simulink model "bike_model_v1_20190513_oldmodel"  (R2016b)
settings: Solver=ode23s  StartTime=0.0  StopTime=sim_time  FixedStep=Ts_IMU  MaxStep=Ts  RelTol=1e-3
values from neighbouring files (symbols this model uses):
  A = [0      0            1 ... (first row only)    [bike_init_v1_20190523_oldmodel_NOfeedback_RealModelComparison.m]    (also in bike_init_v1_20190524_oldmodel_positionfeedback_Nobalancing.m; bike_init_v1_20190527_oldmodel_NObalancing.m; bike_init_v1_20190527_oldmodel_positionfeedback_and_indicator.m; bike_init_v1_20190528_oldmodel_positionfeedback_and_indicator.m)
  B = [0; 1; (a_real*v*sin(lambda_real))/(h_real*b_real)]    [bike_init_v1_20190523_oldmodel_NOfeedback_RealModelComparison.m]    (also in bike_init_v1_20190524_oldmodel_positionfeedback_Nobalancing.m; bike_init_v1_20190527_oldmodel_NObalancing.m; bike_init_v1_20190527_oldmodel_positionfeedback_and_indicator.m; bike_init_v1_20190528_oldmodel_positionfeedback_and_indicator.m)
  b_model = 1.095*(1+(-0.1+(0.2*rand)))    [bike_init_v1_20190523_oldmodel_NOfeedback_RealModelComparison.m]    (also in bike_init_v1_20190524_oldmodel_positionfeedback_Nobalancing.m = 1.095; bike_init_v1_20190527_oldmodel_NObalancing.m = 1.095; bike_init_v1_20190527_oldmodel_positionfeedback_and_indicator.m = 1.095; bike_init_v1_20190528_oldmodel_positionfeedback_and_indicator.m = 1.095)
  b_real = 1.095    [bike_init_v1_20190523_oldmodel_NOfeedback_RealModelComparison.m]    (also in bike_init_v1_20190524_oldmodel_positionfeedback_Nobalancing.m; bike_init_v1_20190527_oldmodel_NObalancing.m; bike_init_v1_20190527_oldmodel_positionfeedback_and_indicator.m; bike_init_v1_20190528_oldmodel_positionfeedback_and_indicator.m)
  complementary = 0.985    [bike_init_v1_20190523_oldmodel_NOfeedback_RealModelComparison.m]    (also in bike_init_v1_20190524_oldmodel_positionfeedback_Nobalancing.m; bike_init_v1_20190527_oldmodel_NObalancing.m; bike_init_v1_20190527_oldmodel_positionfeedback_and_indicator.m; bike_init_v1_20190528_oldmodel_positionfeedback_and_indicator.m)
  cumulative_dist_along_path = [0;cumsum(dist_from_vertex_to_vertex,1)]    [bike_init_v1_20190523_oldmodel_NOfeedback_RealModelComparison.m]    (also in bike_init_v1_20190524_oldmodel_positionfeedback_Nobalancing.m; bike_init_v1_20190527_oldmodel_NObalancing.m; bike_init_v1_20190527_oldmodel_positionfeedback_and_indicator.m; bike_init_v1_20190528_oldmodel_positionfeedback_and_indicator.m)
  damp = 0.4    [bike_init_v1_20190523_oldmodel_NOfeedback_RealModelComparison.m]    (also in bike_init_v1_20190524_oldmodel_positionfeedback_Nobalancing.m; bike_init_v1_20190527_oldmodel_NObalancing.m; bike_init_v1_20190527_oldmodel_positionfeedback_and_indicator.m; bike_init_v1_20190528_oldmodel_positionfeedback_and_indicator.m)
  Dead_Band = [0.055,-0.055,0.005]    [bike_init_v1_20190523_oldmodel_NOfeedback_RealModelComparison.m]    (also in bike_init_v1_20190524_oldmodel_positionfeedback_Nobalancing.m; bike_init_v1_20190527_oldmodel_NObalancing.m; bike_init_v1_20190527_oldmodel_positionfeedback_and_indicator.m; bike_init_v1_20190528_oldmodel_positionfeedback_and_indicator.m)
  delay = 0.045    [bike_init_v1_20190523_oldmodel_NOfeedback_RealModelComparison.m]    (also in bike_init_v1_20190524_oldmodel_positionfeedback_Nobalancing.m; bike_init_v1_20190527_oldmodel_NObalancing.m; bike_init_v1_20190527_oldmodel_positionfeedback_and_indicator.m; bike_init_v1_20190528_oldmodel_positionfeedback_and_indicator.m)
  delta_control = 1    [bike_init_v1_20190523_oldmodel_NOfeedback_RealModelComparison.m]    (also in bike_init_v1_20190524_oldmodel_positionfeedback_Nobalancing.m; bike_init_v1_20190527_oldmodel_NObalancing.m; bike_init_v1_20190527_oldmodel_positionfeedback_and_indicator.m; bike_init_v1_20190528_oldmodel_positionfeedback_and_indicator.m)
  direct_control = 1    [bike_init_v1_20190523_oldmodel_NOfeedback_RealModelComparison.m]    (also in bike_init_v1_20190524_oldmodel_positionfeedback_Nobalancing.m; bike_init_v1_20190527_oldmodel_NObalancing.m; bike_init_v1_20190527_oldmodel_positionfeedback_and_indicator.m; bike_init_v1_20190528_oldmodel_positionfeedback_and_indicator.m)
  filter_model = 1    [bike_init_v1_20190523_oldmodel_NOfeedback_RealModelComparison.m]    (also in bike_init_v1_20190524_oldmodel_positionfeedback_Nobalancing.m; bike_init_v1_20190527_oldmodel_NObalancing.m; bike_init_v1_20190527_oldmodel_positionfeedback_and_indicator.m; bike_init_v1_20190528_oldmodel_positionfeedback_and_indicator.m)
  forward_motor_dynamics = 0    [bike_init_v1_20190523_oldmodel_NOfeedback_RealModelComparison.m]    (also in bike_init_v1_20190524_oldmodel_positionfeedback_Nobalancing.m; bike_init_v1_20190527_oldmodel_NObalancing.m; bike_init_v1_20190527_oldmodel_positionfeedback_and_indicator.m; bike_init_v1_20190528_oldmodel_positionfeedback_and_indicator.m)
  fr_oscil = 1    [bike_init_v1_20190523_oldmodel_NOfeedback_RealModelComparison.m]    (also in bike_init_v1_20190524_oldmodel_positionfeedback_Nobalancing.m; bike_init_v1_20190527_oldmodel_NObalancing.m; bike_init_v1_20190527_oldmodel_positionfeedback_and_indicator.m; bike_init_v1_20190528_oldmodel_positionfeedback_and_indicator.m)
  g = 9.81    [bike_init_v1_20190523_oldmodel_NOfeedback_RealModelComparison.m]    (also in bike_init_v1_20190524_oldmodel_positionfeedback_Nobalancing.m; bike_init_v1_20190527_oldmodel_NObalancing.m; bike_init_v1_20190527_oldmodel_positionfeedback_and_indicator.m; bike_init_v1_20190528_oldmodel_positionfeedback_and_indicator.m)
  gain = 0.3    [bike_init_v1_20190523_oldmodel_NOfeedback_RealModelComparison.m]    (also in bike_init_v1_20190524_oldmodel_positionfeedback_Nobalancing.m; bike_init_v1_20190527_oldmodel_NObalancing.m; bike_init_v1_20190527_oldmodel_positionfeedback_and_indicator.m; bike_init_v1_20190528_oldmodel_positionfeedback_and_indicator.m)
  IMU_height_model = 0.45*(1+(-0.1+(0.2*rand)))    [bike_init_v1_20190523_oldmodel_NOfeedback_RealModelComparison.m]    (also in bike_init_v1_20190524_oldmodel_positionfeedback_Nobalancing.m = 0.45; bike_init_v1_20190527_oldmodel_NObalancing.m = 0.45; bike_init_v1_20190527_oldmodel_positionfeedback_and_indicator.m = 0.45; bike_init_v1_20190528_oldmodel_positionfeedback_and_indicator.m = 0.45)
  IMU_height_real = 0.45    [bike_init_v1_20190523_oldmodel_NOfeedback_RealModelComparison.m]    (also in bike_init_v1_20190524_oldmodel_positionfeedback_Nobalancing.m; bike_init_v1_20190527_oldmodel_NObalancing.m; bike_init_v1_20190527_oldmodel_positionfeedback_and_indicator.m; bike_init_v1_20190528_oldmodel_positionfeedback_and_indicator.m)
  initial_states = [deg2rad(0) deg2rad(0) deg2rad(0)]    [bike_init_v1_20190523_oldmodel_NOfeedback_RealModelComparison.m]    (also in bike_init_v1_20190524_oldmodel_positionfeedback_Nobalancing.m; bike_init_v1_20190527_oldmodel_NObalancing.m; bike_init_v1_20190527_oldmodel_positionfeedback_and_indicator.m; bike_init_v1_20190528_oldmodel_positionfeedback_and_indicator.m = [deg2rad(1) deg2rad(0) deg2rad(0)])
  initial_x = path_x(1)+x_ini_diff    [bike_init_v1_20190523_oldmodel_NOfeedback_RealModelComparison.m]    (also in bike_init_v1_20190524_oldmodel_positionfeedback_Nobalancing.m; bike_init_v1_20190527_oldmodel_NObalancing.m; bike_init_v1_20190527_oldmodel_positionfeedback_and_indicator.m; bike_init_v1_20190528_oldmodel_positionfeedback_and_indicator.m)
  initial_y = radius+y_ini_diff    (= 20)    [bike_init_v1_20190523_oldmodel_NOfeedback_RealModelComparison.m]    (also in bike_init_v1_20190524_oldmodel_positionfeedback_Nobalancing.m; bike_init_v1_20190527_oldmodel_NObalancing.m; bike_init_v1_20190527_oldmodel_positionfeedback_and_indicator.m; bike_init_v1_20190528_oldmodel_positionfeedback_and_indicator.m)
  input_velocity = 2    [bike_init_v1_20190523_oldmodel_NOfeedback_RealModelComparison.m]    (also in bike_init_v1_20190524_oldmodel_positionfeedback_Nobalancing.m = 2.5; bike_init_v1_20190527_oldmodel_NObalancing.m = 2.5; bike_init_v1_20190527_oldmodel_positionfeedback_and_indicator.m = 3; bike_init_v1_20190528_oldmodel_positionfeedback_and_indicator.m = 7)
  K_full_dis = zeros(length(velocity_lqr),3)    [bike_init_v1_20190523_oldmodel_NOfeedback_RealModelComparison.m]    (also in bike_init_v1_20190524_oldmodel_positionfeedback_Nobalancing.m; bike_init_v1_20190527_oldmodel_NObalancing.m; bike_init_v1_20190527_oldmodel_positionfeedback_and_indicator.m; bike_init_v1_20190528_oldmodel_positionfeedback_and_indicator.m)
  lambda_model = deg2rad(70)*(1+(-0.1+(0.2*rand)))    [bike_init_v1_20190523_oldmodel_NOfeedback_RealModelComparison.m]    (also in bike_init_v1_20190524_oldmodel_positionfeedback_Nobalancing.m = deg2rad(70); bike_init_v1_20190527_oldmodel_NObalancing.m = deg2rad(70); bike_init_v1_20190527_oldmodel_positionfeedback_and_indicator.m = deg2rad(70); bike_init_v1_20190528_oldmodel_positionfeedback_and_indicator.m = deg2rad(70))
  lambda_real = deg2rad(70)    [bike_init_v1_20190523_oldmodel_NOfeedback_RealModelComparison.m]    (also in bike_init_v1_20190524_oldmodel_positionfeedback_Nobalancing.m; bike_init_v1_20190527_oldmodel_NObalancing.m; bike_init_v1_20190527_oldmodel_positionfeedback_and_indicator.m; bike_init_v1_20190528_oldmodel_positionfeedback_and_indicator.m)
  lat_control = 1    [bike_init_v1_20190523_oldmodel_NOfeedback_RealModelComparison.m]    (also in bike_init_v1_20190524_oldmodel_positionfeedback_Nobalancing.m; bike_init_v1_20190527_oldmodel_NObalancing.m; bike_init_v1_20190527_oldmodel_positionfeedback_and_indicator.m; bike_init_v1_20190528_oldmodel_positionfeedback_and_indicator.m)
  look_ahead = 0    [bike_init_v1_20190523_oldmodel_NOfeedback_RealModelComparison.m]    (also in bike_init_v1_20190524_oldmodel_positionfeedback_Nobalancing.m; bike_init_v1_20190527_oldmodel_NObalancing.m; bike_init_v1_20190527_oldmodel_positionfeedback_and_indicator.m; bike_init_v1_20190528_oldmodel_positionfeedback_and_indicator.m)
  max_handlebar = 40*(pi/180)    (= 0.698131700798)    [bike_init_v1_20190523_oldmodel_NOfeedback_RealModelComparison.m]    (also in bike_init_v1_20190524_oldmodel_positionfeedback_Nobalancing.m; bike_init_v1_20190527_oldmodel_NObalancing.m; bike_init_v1_20190527_oldmodel_positionfeedback_and_indicator.m; bike_init_v1_20190528_oldmodel_positionfeedback_and_indicator.m)
  max_roll = pi/2    (= 1.57079632679)    [bike_init_v1_20190523_oldmodel_NOfeedback_RealModelComparison.m]    (also in bike_init_v1_20190524_oldmodel_positionfeedback_Nobalancing.m; bike_init_v1_20190527_oldmodel_NObalancing.m; bike_init_v1_20190527_oldmodel_positionfeedback_and_indicator.m; bike_init_v1_20190528_oldmodel_positionfeedback_and_indicator.m)
  max_steering_motor_acc = inf    [bike_init_v1_20190523_oldmodel_NOfeedback_RealModelComparison.m]    (also in bike_init_v1_20190524_oldmodel_positionfeedback_Nobalancing.m; bike_init_v1_20190527_oldmodel_NObalancing.m; bike_init_v1_20190527_oldmodel_positionfeedback_and_indicator.m; bike_init_v1_20190528_oldmodel_positionfeedback_and_indicator.m)
  max_steering_motor_speed = 7.5    [bike_init_v1_20190523_oldmodel_NOfeedback_RealModelComparison.m]    (also in bike_init_v1_20190524_oldmodel_positionfeedback_Nobalancing.m; bike_init_v1_20190527_oldmodel_NObalancing.m; bike_init_v1_20190527_oldmodel_positionfeedback_and_indicator.m; bike_init_v1_20190528_oldmodel_positionfeedback_and_indicator.m)
  min_handlebar = -max_handlebar    (= -0.698131700798)    [bike_init_v1_20190523_oldmodel_NOfeedback_RealModelComparison.m]    (also in bike_init_v1_20190524_oldmodel_positionfeedback_Nobalancing.m; bike_init_v1_20190527_oldmodel_NObalancing.m; bike_init_v1_20190527_oldmodel_positionfeedback_and_indicator.m; bike_init_v1_20190528_oldmodel_positionfeedback_and_indicator.m)
  min_roll = - max_roll    (= -1.57079632679)    [bike_init_v1_20190523_oldmodel_NOfeedback_RealModelComparison.m]    (also in bike_init_v1_20190524_oldmodel_positionfeedback_Nobalancing.m; bike_init_v1_20190527_oldmodel_NObalancing.m; bike_init_v1_20190527_oldmodel_positionfeedback_and_indicator.m; bike_init_v1_20190528_oldmodel_positionfeedback_and_indicator.m)
  min_steering_motor_acc = -inf    [bike_init_v1_20190523_oldmodel_NOfeedback_RealModelComparison.m]    (also in bike_init_v1_20190524_oldmodel_positionfeedback_Nobalancing.m; bike_init_v1_20190527_oldmodel_NObalancing.m; bike_init_v1_20190527_oldmodel_positionfeedback_and_indicator.m; bike_init_v1_20190528_oldmodel_positionfeedback_and_indicator.m)
  min_steering_motor_speed = -7.5    [bike_init_v1_20190523_oldmodel_NOfeedback_RealModelComparison.m]    (also in bike_init_v1_20190524_oldmodel_positionfeedback_Nobalancing.m; bike_init_v1_20190527_oldmodel_NObalancing.m; bike_init_v1_20190527_oldmodel_positionfeedback_and_indicator.m; bike_init_v1_20190528_oldmodel_positionfeedback_and_indicator.m)
  noise = 1    [bike_init_v1_20190523_oldmodel_NOfeedback_RealModelComparison.m]    (also in bike_init_v1_20190524_oldmodel_positionfeedback_Nobalancing.m; bike_init_v1_20190527_oldmodel_NObalancing.m; bike_init_v1_20190527_oldmodel_positionfeedback_and_indicator.m; bike_init_v1_20190528_oldmodel_positionfeedback_and_indicator.m)
  noise_encoder = 1e-7    (= 1e-07)    [bike_init_v1_20190523_oldmodel_NOfeedback_RealModelComparison.m]    (also in bike_init_v1_20190524_oldmodel_positionfeedback_Nobalancing.m; bike_init_v1_20190527_oldmodel_NObalancing.m; bike_init_v1_20190527_oldmodel_positionfeedback_and_indicator.m; bike_init_v1_20190528_oldmodel_positionfeedback_and_indicator.m)
  noise_hall = 0    [bike_init_v1_20190523_oldmodel_NOfeedback_RealModelComparison.m]    (also in bike_init_v1_20190524_oldmodel_positionfeedback_Nobalancing.m = 0.01; bike_init_v1_20190527_oldmodel_NObalancing.m; bike_init_v1_20190527_oldmodel_positionfeedback_and_indicator.m = 0.01; bike_init_v1_20190528_oldmodel_positionfeedback_and_indicator.m = 0.01)
  oscillations_roll = 0    [bike_init_v1_20190523_oldmodel_NOfeedback_RealModelComparison.m]    (also in bike_init_v1_20190524_oldmodel_positionfeedback_Nobalancing.m; bike_init_v1_20190527_oldmodel_NObalancing.m; bike_init_v1_20190527_oldmodel_positionfeedback_and_indicator.m; bike_init_v1_20190528_oldmodel_positionfeedback_and_indicator.m)
  oscillations_steer = 0    [bike_init_v1_20190523_oldmodel_NOfeedback_RealModelComparison.m]    (also in bike_init_v1_20190524_oldmodel_positionfeedback_Nobalancing.m; bike_init_v1_20190527_oldmodel_NObalancing.m; bike_init_v1_20190527_oldmodel_positionfeedback_and_indicator.m; bike_init_v1_20190528_oldmodel_positionfeedback_and_indicator.m)
  parameters_model = [g h_model b_model a_model lambda_model c_model]    [bike_init_v1_20190523_oldmodel_NOfeedback_RealModelComparison.m]    (also in bike_init_v1_20190524_oldmodel_positionfeedback_Nobalancing.m; bike_init_v1_20190527_oldmodel_NObalancing.m; bike_init_v1_20190527_oldmodel_positionfeedback_and_indicator.m; bike_init_v1_20190528_oldmodel_positionfeedback_and_indicator.m)
  parameters_real = [g h_real b_real a_real lambda_real c_real]    [bike_init_v1_20190523_oldmodel_NOfeedback_RealModelComparison.m]    (also in bike_init_v1_20190524_oldmodel_positionfeedback_Nobalancing.m; bike_init_v1_20190527_oldmodel_NObalancing.m; bike_init_v1_20190527_oldmodel_positionfeedback_and_indicator.m; bike_init_v1_20190528_oldmodel_positionfeedback_and_indicator.m)
  path_tracking = 1    [bike_init_v1_20190523_oldmodel_NOfeedback_RealModelComparison.m]    (also in bike_init_v1_20190524_oldmodel_positionfeedback_Nobalancing.m; bike_init_v1_20190527_oldmodel_NObalancing.m; bike_init_v1_20190527_oldmodel_positionfeedback_and_indicator.m; bike_init_v1_20190528_oldmodel_positionfeedback_and_indicator.m = 0)
  path_x = [path_x1 path_x2 path_x3]    [bike_init_v1_20190523_oldmodel_NOfeedback_RealModelComparison.m]    (also in bike_init_v1_20190524_oldmodel_positionfeedback_Nobalancing.m; bike_init_v1_20190527_oldmodel_NObalancing.m; bike_init_v1_20190527_oldmodel_positionfeedback_and_indicator.m; bike_init_v1_20190528_oldmodel_positionfeedback_and_indicator.m)
  path_y = [path_y1 path_y2 path_y3]    [bike_init_v1_20190523_oldmodel_NOfeedback_RealModelComparison.m]    (also in bike_init_v1_20190524_oldmodel_positionfeedback_Nobalancing.m; bike_init_v1_20190527_oldmodel_NObalancing.m; bike_init_v1_20190527_oldmodel_positionfeedback_and_indicator.m; bike_init_v1_20190528_oldmodel_positionfeedback_and_indicator.m)
  plant_model = 1    [bike_init_v1_20190523_oldmodel_NOfeedback_RealModelComparison.m]    (also in bike_init_v1_20190524_oldmodel_positionfeedback_Nobalancing.m; bike_init_v1_20190527_oldmodel_NObalancing.m; bike_init_v1_20190527_oldmodel_positionfeedback_and_indicator.m; bike_init_v1_20190528_oldmodel_positionfeedback_and_indicator.m)
  roll_rate_coef = 0.9    [bike_init_v1_20190523_oldmodel_NOfeedback_RealModelComparison.m]    (also in bike_init_v1_20190524_oldmodel_positionfeedback_Nobalancing.m; bike_init_v1_20190527_oldmodel_NObalancing.m; bike_init_v1_20190527_oldmodel_positionfeedback_and_indicator.m; bike_init_v1_20190528_oldmodel_positionfeedback_and_indicator.m)
  sensordist = dout*pi/nrsensor    (= 0.439822971503)    [bike_init_v1_20190524_oldmodel_positionfeedback_Nobalancing.m]    (also in bike_init_v1_20190527_oldmodel_NObalancing.m; bike_init_v1_20190527_oldmodel_positionfeedback_and_indicator.m; bike_init_v1_20190528_oldmodel_positionfeedback_and_indicator.m; bike_init_v1_20190531_oldmodel_positionfeedback_and_indicator.m)
  steering_motor_limitations = 1    [bike_init_v1_20190523_oldmodel_NOfeedback_RealModelComparison.m]    (also in bike_init_v1_20190524_oldmodel_positionfeedback_Nobalancing.m; bike_init_v1_20190527_oldmodel_NObalancing.m; bike_init_v1_20190527_oldmodel_positionfeedback_and_indicator.m; bike_init_v1_20190528_oldmodel_positionfeedback_and_indicator.m)
  sys_con = ss(A,B,C,D)    [bike_init_v1_20190523_oldmodel_NOfeedback_RealModelComparison.m]    (also in bike_init_v1_20190524_oldmodel_positionfeedback_Nobalancing.m; bike_init_v1_20190527_oldmodel_NObalancing.m; bike_init_v1_20190527_oldmodel_positionfeedback_and_indicator.m; bike_init_v1_20190528_oldmodel_positionfeedback_and_indicator.m)
  sys_dis = c2d(sys_con,Ts)    [bike_init_v1_20190523_oldmodel_NOfeedback_RealModelComparison.m]    (also in bike_init_v1_20190524_oldmodel_positionfeedback_Nobalancing.m; bike_init_v1_20190527_oldmodel_NObalancing.m; bike_init_v1_20190527_oldmodel_positionfeedback_and_indicator.m; bike_init_v1_20190528_oldmodel_positionfeedback_and_indicator.m)
  ToleranceVelocityEst = 0.5    [bike_init_v1_20190524_oldmodel_positionfeedback_Nobalancing.m]    (also in bike_init_v1_20190527_oldmodel_NObalancing.m; bike_init_v1_20190527_oldmodel_positionfeedback_and_indicator.m; bike_init_v1_20190528_oldmodel_positionfeedback_and_indicator.m; bike_init_v1_20190531_oldmodel_positionfeedback_and_indicator.m)
  Ts = 0.04    [bike_init_v1_20190523_oldmodel_NOfeedback_RealModelComparison.m]    (also in bike_init_v1_20190524_oldmodel_positionfeedback_Nobalancing.m; bike_init_v1_20190527_oldmodel_NObalancing.m; bike_init_v1_20190527_oldmodel_positionfeedback_and_indicator.m; bike_init_v1_20190528_oldmodel_positionfeedback_and_indicator.m)
  Ts_IMU = 0.04    [bike_init_v1_20190523_oldmodel_NOfeedback_RealModelComparison.m]    (also in bike_init_v1_20190524_oldmodel_positionfeedback_Nobalancing.m; bike_init_v1_20190527_oldmodel_NObalancing.m; bike_init_v1_20190527_oldmodel_positionfeedback_and_indicator.m; bike_init_v1_20190528_oldmodel_positionfeedback_and_indicator.m)
  velocity_lqr = [velocity_lqr-0.1 velocity_lqr velocity_lqr+0.1]    [bike_init_v1_20190523_oldmodel_NOfeedback_RealModelComparison.m]    (also in bike_init_v1_20190524_oldmodel_positionfeedback_Nobalancing.m; bike_init_v1_20190527_oldmodel_NObalancing.m; bike_init_v1_20190527_oldmodel_positionfeedback_and_indicator.m; bike_init_v1_20190528_oldmodel_positionfeedback_and_indicator.m)
  velocity_wave_amp = 0.5    [bike_init_v1_20190523_oldmodel_NOfeedback_RealModelComparison.m]    (also in bike_init_v1_20190524_oldmodel_positionfeedback_Nobalancing.m; bike_init_v1_20190527_oldmodel_NObalancing.m; bike_init_v1_20190527_oldmodel_positionfeedback_and_indicator.m; bike_init_v1_20190528_oldmodel_positionfeedback_and_indicator.m)
  velocity_wave_freq = 0.3*2*pi    (= 1.88495559215)    [bike_init_v1_20190523_oldmodel_NOfeedback_RealModelComparison.m]    (also in bike_init_v1_20190524_oldmodel_positionfeedback_Nobalancing.m; bike_init_v1_20190527_oldmodel_NObalancing.m; bike_init_v1_20190527_oldmodel_positionfeedback_and_indicator.m; bike_init_v1_20190528_oldmodel_positionfeedback_and_indicator.m)
undefined symbols (not defined in the file or in its folder): curvature
libraries: simulink x13, dspsigops x2, simulink_extras x1
(part 2 of 3)

== system bike_model_v1_20190513_oldmodel/Balance Controller/LQR Controller ==
  note: Input = steering angular velocity
  Velocity : Inport
  State Error : Inport  Port=2
  1-D Lookup Table : Lookup_n-D  NumberOfTableDimensions=1  BreakpointsForDimension1=velocity_lqr  BreakpointsForDimension2=velocity_lqr  BreakpointsForDimension3=velocity_lqr  BreakpointsForDimension4=velocity_lqr  Table=K_full_dis(:,1)  InternalRulePriority=Speed  RndMeth=Simplest  InputSameDT=on
  1-D Lookup Table1 : Lookup_n-D  NumberOfTableDimensions=1  BreakpointsForDimension1=velocity_lqr  BreakpointsForDimension2=velocity_lqr  BreakpointsForDimension3=velocity_lqr  BreakpointsForDimension4=velocity_lqr  Table=K_full_dis(:,2)  InternalRulePriority=Speed  RndMeth=Simplest  InputSameDT=on
  1-D Lookup Table2 : Lookup_n-D  NumberOfTableDimensions=1  BreakpointsForDimension1=velocity_lqr  BreakpointsForDimension2=velocity_lqr  BreakpointsForDimension3=velocity_lqr  BreakpointsForDimension4=velocity_lqr  Table=K_full_dis(:,3)  InternalRulePriority=Speed  RndMeth=Simplest  InputSameDT=on
  Display1 : Display
  Mux : Mux  Inputs=3
  Product : Product  Multiplication=Matrix(*)
  Scope : Scope
  Transpose : Math  Operator=transpose  SaturateOnIntegerOverflow=on
  Zero-Order Hold : ZeroOrderHold  SampleTime=Ts
  Zero-Order Hold1 : ZeroOrderHold  SampleTime=Ts
  Calculated Input : Outport
  wires:
  1-D Lookup Table/1 -> Mux/1  "K1"
  1-D Lookup Table1/1 -> Mux/2  "K2"
  State Error/1 -> Zero-Order Hold1/1
  Product/1 -> Zero-Order Hold/1
  1-D Lookup Table2/1 -> Mux/3  "K3"
  Velocity/1 -> 1-D Lookup Table2/1, 1-D Lookup Table1/1, 1-D Lookup Table/1
  Mux/1 -> Product/2, Display1/1
  Transpose/1 -> Product/1
  Zero-Order Hold/1 -> Calculated Input/1
  Zero-Order Hold1/1 -> Scope/1, Transpose/1

== system bike_model_v1_20190513_oldmodel/Balance Controller/Reference States ==
  Velocity : Inport
  Delta Ref : Inport  Port=2
  Bike Parameters : Constant  Value=parameters_real
  Constant : Constant  Value=path_tracking
  Mux5 : Mux  Inputs=3
  Reference Roll Angle Calculator : MATLAB Function  TreatAsAtomicUnit=on
  Switch : Switch  Criteria=u2 > Threshold
  Reference States : Outport
  wires:
  Bike Parameters/1 -> Reference Roll Angle Calculator/1(parameters_real)
  Switch/1 -> Mux5/2, Reference Roll Angle Calculator/3(delta_ref)
  Reference Roll Angle Calculator/1(phi_ref) -> Mux5/1
  Velocity/1 -> Reference Roll Angle Calculator/2(velocity)
  Mux5/1 -> Reference States/1
  Constant/1 -> Switch/2
  Delta Ref/1 -> Switch/1

== system bike_model_v1_20190513_oldmodel/Complementary filter/Complementary Filter ==
  Roll Angle Estimation due to Accelerometer : Inport
  Roll Rate due to Gyroscope : Inport  Port=2
  Delay : Delay  DelayLength=1  InitialCondition=0
  Gain2 : Gain  Gain=complementary
  Gain3 : Gain  Gain=1-complementary
  Gain4 : Gain  Gain=Ts_IMU
  Sum3 : Sum  Inputs=|++
  Sum4 : Sum  Inputs=++|
  Roll Angle Estimation : Outport
  wires:
  Roll Angle Estimation due to Accelerometer/1 -> Gain3/1  "Roll_acc"
  Sum3/1 -> Gain2/1
  Roll Rate due to Gyroscope/1 -> Gain4/1
  Delay/1 -> Sum3/2
  Gain4/1 -> Sum3/1
  Gain2/1 -> Sum4/2
  Gain3/1 -> Sum4/1
  Sum4/1 -> Delay/1, Roll Angle Estimation/1

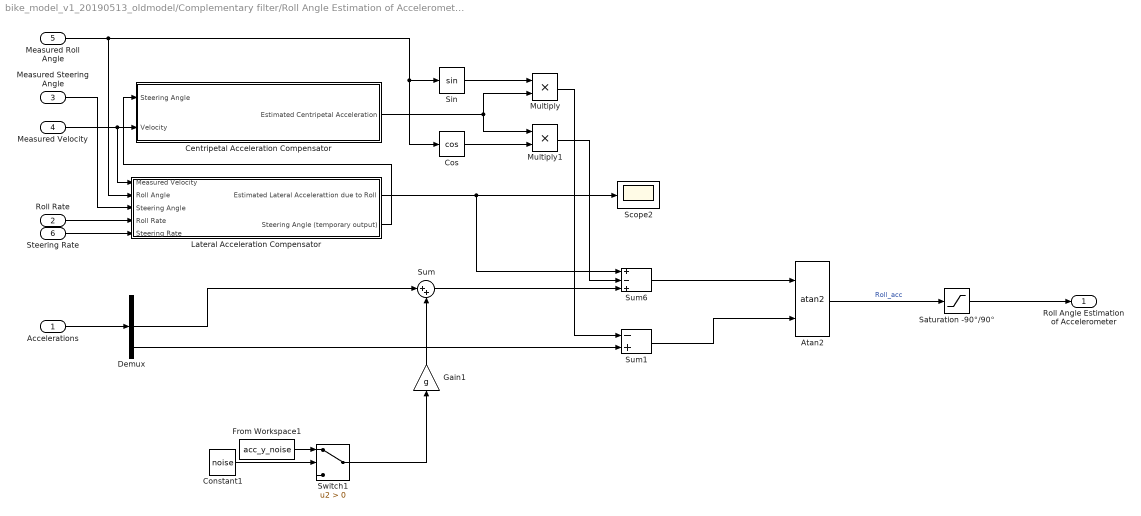
== system bike_model_v1_20190513_oldmodel/Complementary filter/Roll Angle Estimation of Accelerometer ==
  Accelerations : Inport
  Roll Rate : Inport  Port=2
  Measured Steering Angle : Inport  Port=3
  Measured Velocity : Inport  Port=4
  Measured Roll Angle : Inport  Port=5
  Steering Rate : Inport  Port=6
  Atan2 : Trigonometry  Operator=atan2
  Centripetal Acceleration Compensator : Subsystem
  Constant1 : Constant  Value=noise
  Cos : Trigonometry  Operator=cos
  Demux : Demux  Outputs=3
  From Workspace1 : FromWorkspace  VariableName=acc_y_noise  SampleTime=0
  Gain1 : Gain  Gain=g
  Lateral Acceleration Compensator : Subsystem
  Multiply : Product
  Multiply1 : Product
  Saturation -90°/90° : Saturate  UpperLimit=max_roll  LowerLimit=min_roll
  Scope2 : Scope
  Sin : Trigonometry
  Sum : Sum  Inputs=|++
  Sum1 : Sum  Inputs=-+
  Sum6 : Sum  Inputs=+-+
  Switch1 : Switch  Criteria=u2 > Threshold
  Roll Angle Estimation of Accelerometer : Outport
  wires:
  Sum1/1 -> Atan2/2
  Lateral Acceleration Compensator/1(Estimated Lateral Accelerattion due to Roll) -> Scope2/1, Sum6/1
  Atan2/1 -> Saturation -90°/90°/1  "Roll_acc"
  Roll Rate/1 -> Lateral Acceleration Compensator/4(Roll Rate)
  Demux/2 -> Sum/1
  Accelerations/1 -> Demux/1
  Measured Velocity/1 -> Lateral Acceleration Compensator/1(Measured Velocity), Centripetal Acceleration Compensator/2(Velocity)
  Measured Steering Angle/1 -> Lateral Acceleration Compensator/3(Steering Angle)
  Centripetal Acceleration Compensator/1(Estimated Centripetal Acceleration) -> Multiply/2, Multiply1/1
  Measured Roll Angle/1 -> Lateral Acceleration Compensator/2(Roll Angle), Sin/1, Cos/1
  Cos/1 -> Multiply1/2
  Sin/1 -> Multiply/1
  Multiply1/1 -> Sum6/2
  Demux/3 -> Sum1/2
  Multiply/1 -> Sum1/1
  Steering Rate/1 -> Lateral Acceleration Compensator/5(Steering Rate)
  Sum6/1 -> Atan2/1
  Lateral Acceleration Compensator/2(Steering Angle (temporary output)) -> Centripetal Acceleration Compensator/1(Steering Angle)
  From Workspace1/1 -> Switch1/1
  Constant1/1 -> Switch1/2
  Sum/1 -> Sum6/3
  Switch1/1 -> Gain1/1
  Gain1/1 -> Sum/2
  Saturation -90°/90°/1 -> Roll Angle Estimation of Accelerometer/1

== system bike_model_v1_20190513_oldmodel/Global Angles and Coordinates Calculator/Measured Bike Angles to Global Angles ==
  Velocity : Inport
  Steering Angle : Inport  Port=2
  Gain : Gain  Gain=1/b_model
  Integrator : Integrator
  MATLAB Function : MATLAB Function  TreatAsAtomicUnit=on
  Multiply : Product
  Parameters : Constant  Value=parameters_model
  Scope : Scope  NumInputPorts=2
  Tan : Trigonometry  Operator=tan
  psi : Outport
  beta : Outport  Port=2
  wires:
  Integrator/1 -> psi/1
  MATLAB Function/1(psi_d) -> Scope/1, Integrator/1
  Steering Angle/1 -> Tan/1, MATLAB Function/3(delta)
  Parameters/1 -> MATLAB Function/2(parameters_model)
  Velocity/1 -> Multiply/1, MATLAB Function/1(v)
  MATLAB Function/2(beta) -> beta/1
  Tan/1 -> Multiply/2
  Multiply/1 -> Gain/1
  Gain/1 -> Scope/2

== system bike_model_v1_20190513_oldmodel/Global Angles and Coordinates Calculator/Measured Global Angles to Global Coordinates ==
  Velocity : Inport
  Psi : Inport  Port=2
  Beta : Inport  Port=3
  Constant : Constant  Value=initial_y
  Constant1 : Constant  Value=initial_x
  Integrator1 : Integrator
  Integrator2 : Integrator
  MATLAB Function1 : MATLAB Function  TreatAsAtomicUnit=on
  Mux : Mux  Inputs=2
  Sum : Sum  Inputs=|++
  Sum1 : Sum  Inputs=++|
  "Position (X, Y)" : Outport
  wires:
  MATLAB Function1/2(Ydot) -> Integrator2/1  "Ydot"
  MATLAB Function1/1(Xdot) -> Integrator1/1  "Xdot"
  Psi/1 -> MATLAB Function1/2(psi)
  Beta/1 -> MATLAB Function1/3(beta)
  Velocity/1 -> MATLAB Function1/1(v)
  Integrator2/1 -> Sum/1
  Constant/1 -> Sum/2
  Sum/1 -> Mux/2
  Integrator1/1 -> Sum1/2
  Sum1/1 -> Mux/1
  Constant1/1 -> Sum1/1
  Mux/1 -> "Position (X, Y)"/1

== system bike_model_v1_20190513_oldmodel/Global Angles and Coordinates Calculator/Path Plotter Reality ==
  Position : Inport
  Demux : Demux  Outputs=2
  To Workspace : ToWorkspace  VariableName=X_BIKE  SaveFormat=Timeseries  SampleTime=Ts
  To Workspace1 : ToWorkspace  VariableName=Y_BIKE  SaveFormat=Timeseries  SampleTime=Ts
  XY Graph : simulink/Sinks/XY Graph  Commented=on  xmin=min(path_x)-5  xmax=max(path_x)+5  ymin=min(path_y)-5  ymax=max(path_y)+5  st=-1
  wires:
  Demux/1 -> XY Graph/1, To Workspace/1  "X"
  Demux/2 -> XY Graph/2, To Workspace1/1  "Y"
  Position/1 -> Demux/1

== system bike_model_v1_20190513_oldmodel/Global Angles and Coordinates Calculator/Path Plotter estimation ==
  Position : Inport
  Demux : Demux  Outputs=2
  To Workspace : ToWorkspace  VariableName=X_BIKE_estim  SaveFormat=Timeseries  SampleTime=Ts
  To Workspace1 : ToWorkspace  VariableName=Y_BIKE_estim  SaveFormat=Timeseries  SampleTime=Ts
  XY Graph : simulink/Sinks/XY Graph  Commented=on  xmin=min(path_x)-5  xmax=max(path_x)+5  ymin=min(path_y)-5  ymax=max(path_y)+5  st=-1
  wires:
  Demux/1 -> XY Graph/1, To Workspace/1  "X"
  Demux/2 -> XY Graph/2, To Workspace1/1  "Y"
  Position/1 -> Demux/1

== system bike_model_v1_20190513_oldmodel/Global Angles and Coordinates Calculator/True Bike Angles to Global Angles2 ==
  Velocity : Inport
  Steering Angle : Inport  Port=2
  Integrator : Integrator
  MATLAB Function : MATLAB Function  TreatAsAtomicUnit=on
  Real Bike Parameters : Constant  Value=parameters_real
  To Workspace6 : ToWorkspace  VariableName=PSI  SaveFormat=Timeseries  SampleTime=Ts
  To Workspace7 : ToWorkspace  VariableName=BETA  SaveFormat=Timeseries  SampleTime=Ts
  psi : Outport
  beta : Outport  Port=2
  wires:
  Integrator/1 -> To Workspace6/1, psi/1
  MATLAB Function/1(psi_d) -> Integrator/1
  Steering Angle/1 -> MATLAB Function/3(delta)
  Real Bike Parameters/1 -> MATLAB Function/2(parameters_real)
  Velocity/1 -> MATLAB Function/1(v)
  MATLAB Function/2(beta) -> beta/1, To Workspace7/1

== system bike_model_v1_20190513_oldmodel/Global Angles and Coordinates Calculator/True Global Angles to Global Coordinates ==
  Velocity : Inport
  Psi : Inport  Port=2
  Beta : Inport  Port=3
  Constant : Constant  Value=initial_y
  Constant1 : Constant  Value=initial_x
  Integrator1 : Integrator
  Integrator2 : Integrator
  MATLAB Function1 : MATLAB Function  TreatAsAtomicUnit=on
  Mux : Mux  Inputs=2
  Sum : Sum  Inputs=|++
  Sum1 : Sum  Inputs=++|
  "Position (X, Y)" : Outport
  wires:
  MATLAB Function1/2(Ydot) -> Integrator2/1  "Ydot"
  MATLAB Function1/1(Xdot) -> Integrator1/1  "Xdot"
  Psi/1 -> MATLAB Function1/2(psi)
  Beta/1 -> MATLAB Function1/3(beta)
  Velocity/1 -> MATLAB Function1/1(v)
  Integrator2/1 -> Sum/1
  Constant/1 -> Sum/2
  Sum/1 -> Mux/2
  Integrator1/1 -> Sum1/2
  Sum1/1 -> Mux/1
  Constant1/1 -> Sum1/1
  Mux/1 -> "Position (X, Y)"/1

== system bike_model_v1_20190513_oldmodel/IMU/IMU ==
  Lateral Acceleration : Inport
  Centripetal Acceleration : Inport  Port=2
  True Velocity : Inport  Port=3
  True Roll Angle : Inport  Port=4
  Measured Steering Angle : Inport  Port=5
  IMU Accelerometer : Subsystem
  IMU Gyroscope : Subsystem
  Accelerations : Outport
  Roll Rates : Outport  Port=2
  wires:
  Lateral Acceleration/1 -> IMU Accelerometer/1(Lateral Acceleration of the IMU due to Roll)
  Centripetal Acceleration/1 -> IMU Accelerometer/2(Centripetal Acceleration due to Path Curvature)
  True Roll Angle/1 -> IMU Gyroscope/2(True Roll Angle), IMU Accelerometer/4(True Roll Angle)
  IMU Accelerometer/1(Accelerations) -> Accelerations/1
  IMU Gyroscope/1(Roll rates) -> Roll Rates/1
  True Velocity/1 -> IMU Gyroscope/1(True Velocity), IMU Accelerometer/3(True Velocity)
  Measured Steering Angle/1 -> IMU Gyroscope/3(Measured Steering Angle)

== system bike_model_v1_20190513_oldmodel/Path Tracking Controllers/Lateral Error ==
  Psi Sigma : Inport
  Position Error (X,Y) : Inport  Port=2
  Cos : Trigonometry  Operator=cos
  Demux : Demux  Outputs=2
  Product : Product
  Product1 : Product
  Sin : Trigonometry
  Sum : Sum  Inputs=+-|
  To Workspace4 : ToWorkspace  VariableName=LAT_ERR  SaveFormat=Timeseries  SampleTime=Ts
  Lateral Error : Outport
  wires:
  Cos/1 -> Product/2
  Sin/1 -> Product1/1
  Psi Sigma/1 -> Cos/1, Sin/1
  Product1/1 -> Sum/2
  Product/1 -> Sum/1
  Sum/1 -> To Workspace4/1, Lateral Error/1  "Lateral Error"
  Demux/1 -> Product1/2  "X Position Error"
  Demux/2 -> Product/1  "Y Position Error"
  Position Error (X,Y)/1 -> Demux/1

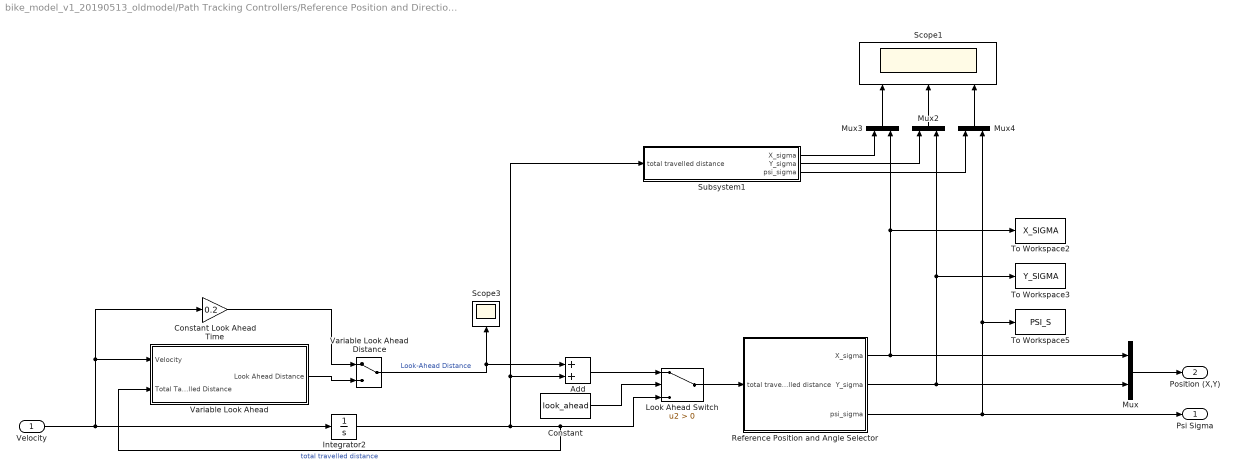
== system bike_model_v1_20190513_oldmodel/Path Tracking Controllers/Reference Position and Direction in Global CS with variable Look Ahead ==
  Velocity : Inport
  Add : Sum
  Constant : Constant  Value=look_ahead
  Constant Look Ahead Time : Gain  Gain=0.2
  Integrator2 : Integrator
  Look Ahead Switch : Switch  Criteria=u2 > Threshold
  Mux{,2..4} (4 alike) : Mux  Inputs=2
  Reference Position and Angle Selector : Subsystem
  Scope1 : Scope  NumInputPorts=3
  Scope3 : Scope
  Subsystem1 : Subsystem
  To Workspace2 : ToWorkspace  VariableName=X_SIGMA  SaveFormat=Timeseries  SampleTime=Ts
  To Workspace3 : ToWorkspace  VariableName=Y_SIGMA  SaveFormat=Timeseries  SampleTime=Ts
  To Workspace5 : ToWorkspace  VariableName=PSI_S  SaveFormat=Timeseries  SampleTime=Ts
  Variable Look Ahead Distance : ManualSwitch
  Variable Look Ahead : Subsystem
  Psi Sigma : Outport
  Position (X,Y) : Outport  Port=2
  wires:
  Constant Look Ahead Time/1 -> Variable Look Ahead Distance/1
  Reference Position and Angle Selector/3(psi_sigma) -> To Workspace5/1, Mux4/2, Psi Sigma/1
  Mux3/1 -> Scope1/1
  Subsystem1/3(psi_sigma) -> Mux4/1
  Mux2/1 -> Scope1/2
  Mux4/1 -> Scope1/3
  Velocity/1 -> Integrator2/1, Constant Look Ahead Time/1, Variable Look Ahead/1(Velocity)
  Add/1 -> Look Ahead Switch/1
  Reference Position and Angle Selector/2(Y_sigma) -> To Workspace3/1, Mux2/2, Mux/2
  Look Ahead Switch/1 -> Reference Position and Angle Selector/1(total travelled distance)
  Subsystem1/2(Y_sigma) -> Mux2/1
  Integrator2/1 -> Variable Look Ahead/2(Total Tavelled Distance), Look Ahead Switch/3, Subsystem1/1(total travelled distance), Add/2  "total travelled distance"
  Subsystem1/1(X_sigma) -> Mux3/1
  Reference Position and Angle Selector/1(X_sigma) -> Mux3/2, To Workspace2/1, Mux/1
  Variable Look Ahead Distance/1 -> Scope3/1, Add/1  "Look-Ahead Distance"
  Constant/1 -> Look Ahead Switch/2
  Mux/1 -> Position (X,Y)/1
  Variable Look Ahead/1(Look Ahead Distance) -> Variable Look Ahead Distance/2

== system bike_model_v1_20190513_oldmodel/Physical Bike/Centripetal Acceleration Calculator ==
  True Steering Angle : Inport
  True Velocity : Inport  Port=2
  Divide : Product  Inputs=*/
  Gain : Gain  Gain=sin(lambda_real)
  Multiply : Product
  Square : Math  Operator=square  SaturateOnIntegerOverflow=on
  Tan : Trigonometry  Operator=tan
  b Real Bike : Constant  Value=b_real
  Centripetal Acceleration : Outport
  wires:
  True Velocity/1 -> Square/1
  Square/1 -> Divide/1
  b Real Bike/1 -> Divide/2
  True Steering Angle/1 -> Gain/1
  Divide/1 -> Multiply/1
  Tan/1 -> Multiply/2
  Multiply/1 -> Centripetal Acceleration/1
  Gain/1 -> Tan/1

== system bike_model_v1_20190513_oldmodel/Physical Bike/Check Phi Limits ==
  x : Inport
  Roll Lower Bound : simulink/Model Verification/Check Static  Lower Bound  Description=min_roll <= u  min=min_roll  min_included=on  enabled=on  stopWhenAssertionFail=on  export=off  icon=graphic
  Roll Upper Bound : simulink/Model Verification/Check Static  Upper Bound  Description=u <= max_roll  max=max_roll  max_included=on  enabled=on  stopWhenAssertionFail=on  export=off  icon=graphic
  wires:
  x/1 -> Roll Lower Bound/1, Roll Upper Bound/1  "Roll Angle"

== system bike_model_v1_20190513_oldmodel/Physical Bike/Lateral Acceleration (due to Roll) Calculator ==
  Roll Acceleration : Inport
  Constant3 : Constant  Value=IMU_height_real
  Multiply : Product
  Lateral Acceleration : Outport
  wires:
  Multiply/1 -> Lateral Acceleration/1
  Constant3/1 -> Multiply/1
  Roll Acceleration/1 -> Multiply/2

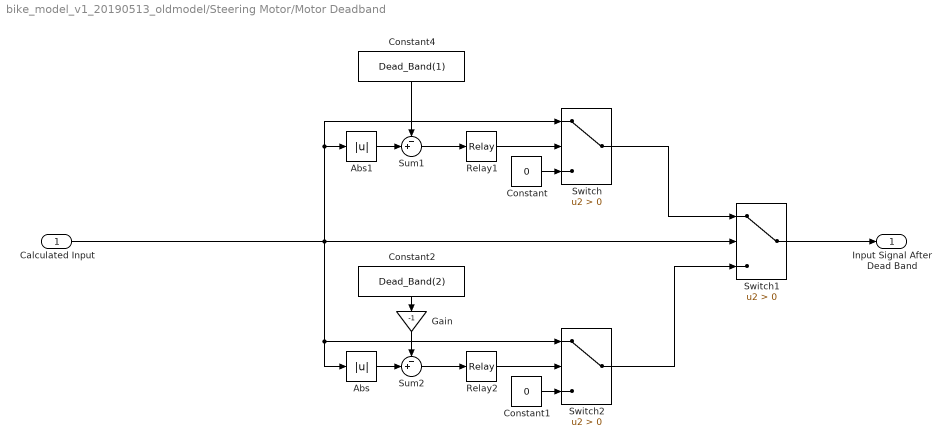
== system bike_model_v1_20190513_oldmodel/Steering Motor/Motor Deadband ==
  Calculated Input : Inport
  Abs : Abs
  Abs1 : Abs
  Constant : Constant  Value=0  SampleTime=Ts
  Constant1 : Constant  Value=0  SampleTime=Ts
  Constant2 : Constant  Value=Dead_Band(2)  SampleTime=Ts
  Constant4 : Constant  Value=Dead_Band(1)  SampleTime=Ts
  Gain : Gain  Gain=-1
  Relay1 : Relay  OnSwitchValue=Dead_Band(3)  OffSwitchValue=-Dead_Band(3)
  Relay2 : Relay  OnSwitchValue=Dead_Band(3)  OffSwitchValue=-Dead_Band(3)
  Sum1 : Sum  Inputs=-+|
  Sum2 : Sum  Inputs=-+|
  Switch : Switch  Criteria=u2 > Threshold
  Switch1 : Switch  Criteria=u2 > Threshold
  Switch2 : Switch  Criteria=u2 > Threshold
  Input Signal After Dead Band : Outport
  wires:
  Constant4/1 -> Sum1/1
  Sum1/1 -> Relay1/1
  Relay1/1 -> Switch/2
  Switch/1 -> Switch1/1
  Constant/1 -> Switch/3
  Switch1/1 -> Input Signal After Dead Band/1
  Switch2/1 -> Switch1/3
  Constant1/1 -> Switch2/3
  Gain/1 -> Sum2/1
  Calculated Input/1 -> Abs/1, Switch2/1, Abs1/1, Switch/1, Switch1/2
  Sum2/1 -> Relay2/1
  Relay2/1 -> Switch2/2
  Abs/1 -> Sum2/2
  Abs1/1 -> Sum1/2
  Constant2/1 -> Gain/1

== system bike_model_v1_20190513_oldmodel/Steering Motor/Velocity Saturation wrt Max and Min Handle Bar Angles ==
  Reference Velocity : Inport
  States : Inport  Port=2
  AND : Logic  IconShape=distinctive  AllPortsSameDT=off  OutDataTypeStr=boolean
  AND1 : Logic  IconShape=distinctive  AllPortsSameDT=off  OutDataTypeStr=boolean
  Compare To Constant : simulink/Logic and Bit Operations/Compare To Constant  relop=>=  const=max_handlebar  OutDataTypeStr=boolean
  Compare To Constant1 : simulink/Logic and Bit Operations/Compare To Constant  relop=<=  const=min_handlebar  OutDataTypeStr=boolean
  Compare To Zero : simulink/Logic and Bit Operations/Compare To Zero  relop=>=  OutDataTypeStr=boolean
  Compare To Zero1 : simulink/Logic and Bit Operations/Compare To Zero  relop=<=  OutDataTypeStr=boolean
  Constant : Constant  Value=0
  Demux : Demux  Outputs=3
  OR : Logic  Operator=OR  IconShape=distinctive  AllPortsSameDT=off  OutDataTypeStr=boolean
  Switch : Switch  Criteria=u2 > Threshold
  Output Steering Velocity : Outport
  wires:
  Switch/1 -> Output Steering Velocity/1
  Constant/1 -> Switch/1
  States/1 -> Demux/1
  Compare To Zero/1 -> AND/1
  Compare To Zero1/1 -> AND1/2
  Demux/2 -> Compare To Constant/1, Compare To Constant1/1
  Compare To Constant1/1 -> AND1/1
  AND/1 -> OR/1
  AND1/1 -> OR/2
  Compare To Constant/1 -> AND/2
  Reference Velocity/1 -> Compare To Zero1/1, Compare To Zero/1, Switch/3
  OR/1 -> Switch/2

== system bike_model_v1_20190513_oldmodel/Complementary filter/Roll Angle Estimation of Accelerometer/Centripetal Acceleration Compensator ==
  Steering Angle : Inport
  Velocity : Inport  Port=2
  Bike Model b : Constant  Value=b_model
  Divide : Product  Inputs=*/
  Gain : Gain  Gain=sin(lambda_model)
  Multiply : Product
  Square : Math  Operator=square  SaturateOnIntegerOverflow=on
  Tan : Trigonometry  Operator=tan
  Estimated Centripetal Acceleration : Outport
  wires:
  Velocity/1 -> Square/1
  Square/1 -> Divide/1
  Bike Model b/1 -> Divide/2
  Steering Angle/1 -> Gain/1
  Divide/1 -> Multiply/1
  Tan/1 -> Multiply/2
  Multiply/1 -> Estimated Centripetal Acceleration/1
  Gain/1 -> Tan/1

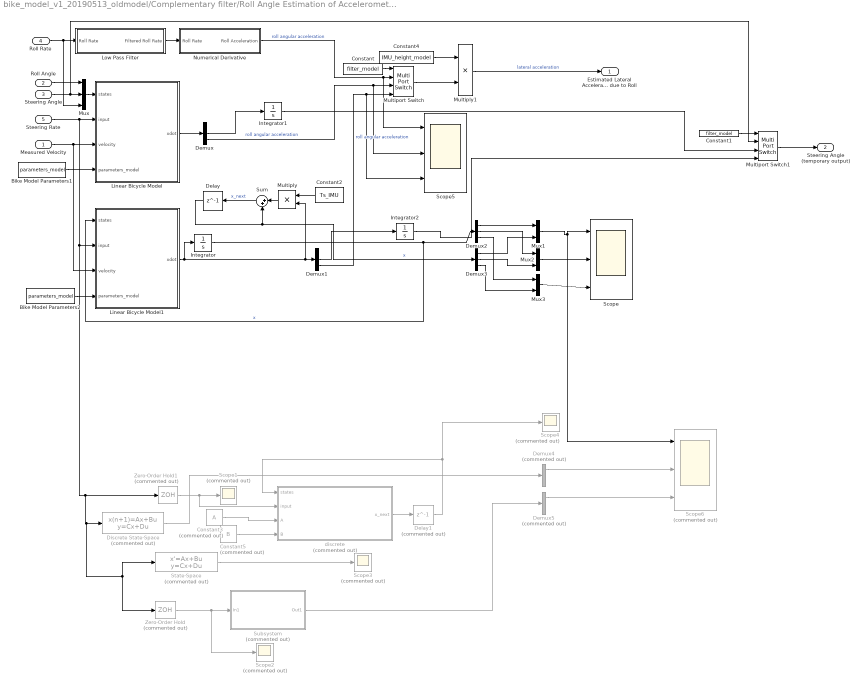
== system bike_model_v1_20190513_oldmodel/Complementary filter/Roll Angle Estimation of Accelerometer/Lateral Acceleration Compensator ==
  Measured Velocity : Inport
  Roll Angle : Inport  Port=2
  Steering Angle : Inport  Port=3
  Roll Rate : Inport  Port=4
  Steering Rate : Inport  Port=5
  Bike Model Parameters1 : Constant  Value=parameters_model
  Bike Model Parameters2 : Constant  Value=parameters_model
  Constant : Constant  Value=filter_model
  Constant1 : Constant  Value=filter_model
  Constant2 : Constant  Value=Ts_IMU  SampleTime=Ts_IMU
  Constant3 : Constant  Commented=on  Value=A
  Constant4 : Constant  Value=IMU_height_model
  Constant5 : Constant  Commented=on  Value=B
  Delay : Delay  DelayLength=1  InitialCondition=[0 0 0]  SampleTime=Ts_IMU
  Delay1 : Delay  Commented=on  DelayLength=1  InitialCondition=[0 0 0]  SampleTime=Ts_IMU
  Demux{,1..3} (4 alike) : Demux  Outputs=3
  Demux4 : Demux  Commented=on  Outputs=3
  Demux5 : Demux  Commented=on  Outputs=3
  Discrete State-Space : DiscreteStateSpace  Commented=on  A=A  B=B  C=eye(3,3)  D=zeros(3,1)  X0=[0 0 0]  SampleTime=Ts_IMU
  Integrator : Integrator  InitialCondition=initial_states
  Integrator1 : Integrator  InitialCondition=initial_states(2)
  Integrator2 : Integrator  InitialCondition=initial_states(2)
  Linear Bicycle Model : MATLAB Function  TreatAsAtomicUnit=on
  Linear Bicycle Model1 : MATLAB Function  TreatAsAtomicUnit=on
  Low Pass Filter : Subsystem
  Multiply : Product
  Multiply1 : Product
  Multiport Switch : MultiPortSwitch
  Multiport Switch1 : MultiPortSwitch
  Mux : Mux  Inputs=3
  Mux1 : Mux  Inputs=2
  Mux2 : Mux  Inputs=2
  Mux3 : Mux  Inputs=2
  Numerical Derivative : Subsystem
  Scope : Scope  NumInputPorts=3
  Scope{1..4} (4 alike) : Scope  Commented=on
  Scope5 : Scope  NumInputPorts=3
  Scope6 : Scope  Commented=on  NumInputPorts=3
  State-Space : StateSpace  Commented=on  A=sys_con.A  B=sys_con.B  C=eye(3,3)  D=zeros(3,1)  X0=[0 0 0]
  Subsystem : Subsystem  Commented=on  TreatAsAtomicUnit=on  SystemSampleTime=Ts_IMU
  Sum : Sum  Inputs=|++
  Zero-Order Hold : ZeroOrderHold  Commented=on  SampleTime=Ts_IMU
  Zero-Order Hold1 : ZeroOrderHold  Commented=on  SampleTime=Ts_IMU
  discrete : MATLAB Function  Commented=on  TreatAsAtomicUnit=on
  Estimated Lateral Accelerattion due to Roll : Outport
  Steering Angle (temporary output) : Outport  Port=2
  wires:
  Numerical Derivative/1(Roll Acceleration) -> Scope5/1, Multiport Switch/2  "roll angular acceleration"
  Roll Rate/1 -> Mux/3, Low Pass Filter/1(Roll Rate)
  Constant4/1 -> Multiply1/1
  Multiply1/1 -> Estimated Lateral Accelerattion due to Roll/1  "lateral acceleration"
  Low Pass Filter/1(Filtered Roll Rate) -> Numerical Derivative/1(Roll Rate)
  Linear Bicycle Model/1(xdot) -> Demux/1
  Demux/3 -> Scope5/2, Multiport Switch/3  "roll angular acceleration"
  Bike Model Parameters1/1 -> Linear Bicycle Model/4(parameters_model)
  Measured Velocity/1 -> Linear Bicycle Model1/3(velocity), Linear Bicycle Model/3(velocity)
  Mux/1 -> Linear Bicycle Model/1(states)
  Roll Angle/1 -> Mux/1
  Steering Angle/1 -> Multiport Switch1/2, Mux/2
  Constant/1 -> Multiport Switch/1
  Multiport Switch/1 -> Multiply1/2
  Demux1/3 -> Scope5/3, Multiport Switch/4  "roll angular acceleration"
  Bike Model Parameters2/1 -> Linear Bicycle Model1/4(parameters_model)
  Delay/1 -> Demux3/1, Sum/2  "x"
  Multiply/1 -> Sum/1
  Constant2/1 -> Multiply/1
  Integrator/1 -> Linear Bicycle Model1/1(states), Demux2/1  "x"
  Demux2/1 -> Mux1/1
  Demux3/1 -> Mux1/2
  Demux2/2 -> Mux2/1
  Demux3/2 -> Mux2/2
  Demux2/3 -> Mux3/1
  Demux3/3 -> Mux3/2
  Mux2/1 -> Scope/2
  Mux1/1 -> Scope6/1, Scope/1
  Mux3/1 -> Scope/3
  Linear Bicycle Model1/1(xdot) -> Multiply/2, Demux1/1, Integrator/1
  State-Space/1 -> Scope3/1
  Delay1/1 -> Scope4/1, discrete/1(states)
  Zero-Order Hold/1 -> Scope2/1, Subsystem/1(In1)
  discrete/1(x_next) -> Delay1/1
  Constant5/1 -> discrete/4(B)
  Constant3/1 -> discrete/3(A)
  Sum/1 -> Delay/1  "x_next"
  Zero-Order Hold1/1 -> discrete/2(input), Scope1/1
  Multiport Switch1/1 -> Steering Angle (temporary output)/1
  Constant1/1 -> Multiport Switch1/1
  Steering Rate/1 -> Zero-Order Hold/1, State-Space/1, Discrete State-Space/1, Zero-Order Hold1/1, Linear Bicycle Model1/2(input), Linear Bicycle Model/2(input)
  Integrator1/1 -> Multiport Switch1/3
  Demux/2 -> Integrator1/1
  Demux1/2 -> Integrator2/1
  Integrator2/1 -> Multiport Switch1/4
  Demux4/1 -> Scope6/2
  Demux5/1 -> Scope6/3
  Discrete State-Space/1 -> Demux4/1
  Subsystem/1(Out1) -> Demux5/1

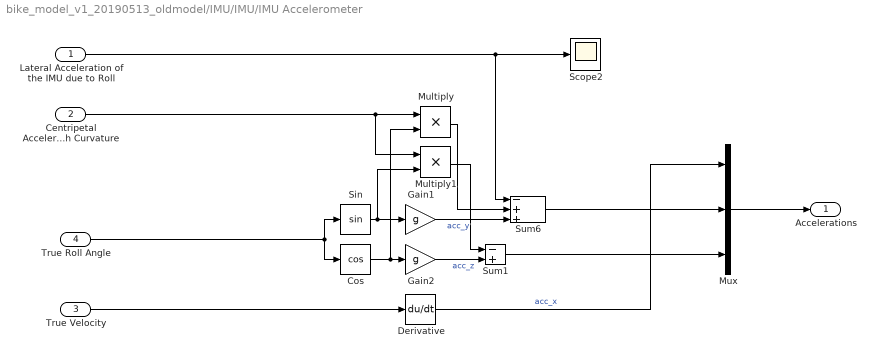
== system bike_model_v1_20190513_oldmodel/IMU/IMU/IMU Accelerometer ==
  Lateral Acceleration of the IMU due to Roll : Inport
  Centripetal Acceleration due to Path Curvature : Inport  Port=2
  True Velocity : Inport  Port=3
  True Roll Angle : Inport  Port=4
  Cos : Trigonometry  Operator=cos
  Derivative : Derivative  CoefficientInTFapproximation=-1
  Gain1 : Gain  Gain=g
  Gain2 : Gain  Gain=g
  Multiply : Product
  Multiply1 : Product
  Mux : Mux  Inputs=3
  Scope2 : Scope
  Sin : Trigonometry
  Sum1 : Sum  Inputs=-+
  Sum6 : Sum  Inputs=-++
  Accelerations : Outport
  wires:
  Multiply/1 -> Sum6/2
  Gain1/1 -> Sum6/3  "acc_y"
  Sin/1 -> Multiply1/2, Gain1/1
  Derivative/1 -> Mux/1  "acc_x"
  Cos/1 -> Multiply/2, Gain2/1
  Gain2/1 -> Sum1/2  "acc_z"
  True Roll Angle/1 -> Sin/1, Cos/1
  True Velocity/1 -> Derivative/1
  Centripetal Acceleration due to Path Curvature/1 -> Multiply1/1, Multiply/1
  Multiply1/1 -> Sum1/1
  Sum1/1 -> Mux/3
  Mux/1 -> Accelerations/1
  Sum6/1 -> Mux/2
  Lateral Acceleration of the IMU due to Roll/1 -> Sum6/1, Scope2/1

== system bike_model_v1_20190513_oldmodel/IMU/IMU/IMU Gyroscope ==
  True Velocity : Inport
  True Roll Angle : Inport  Port=2
  Measured Steering Angle : Inport  Port=3
  "Bike Model b " : Constant  Value=b_model
  Cos : Trigonometry  Operator=cos
  Divide : Product  Inputs=*/
  Gain : Gain  Gain=sin(lambda_model)
  Multiply : Product
  Multiply1 : Product
  Multiply2 : Product
  Mux : Mux  Inputs=3
  Sin : Trigonometry
  Tan : Trigonometry  Operator=tan
  Roll rates : Outport
  wires:
  Mux/1 -> Roll rates/1
  Tan/1 -> Multiply/1
  Gain/1 -> Tan/1
  Measured Steering Angle/1 -> Gain/1
  Cos/1 -> Multiply1/1
  True Roll Angle/1 -> Mux/1, Cos/1, Sin/1
  Sin/1 -> Multiply2/1
  True Velocity/1 -> Divide/1
  "Bike Model b "/1 -> Divide/2
  Divide/1 -> Multiply/2  "v/b"
  Multiply/1 -> Multiply2/2, Multiply1/2
  Multiply2/1 -> Mux/2
  Multiply1/1 -> Mux/3

== system bike_model_v1_20190513_oldmodel/Path Tracking Controllers/Reference Position and Direction in Global CS with variable Look Ahead/Reference Position and Angle Selector ==
  total travelled distance : Inport
  1-D Lookup Table : Lookup_n-D  NumberOfTableDimensions=1  BreakpointsForDimension1=cumulative_dist_along_path  Table=path_x  ExtrapMethod=Clip  DiagnosticForOutOfRangeInput=Error  InternalRulePriority=Speed  RndMeth=Simplest  InputSameDT=on
  1-D Lookup Table1 : Lookup_n-D  NumberOfTableDimensions=1  BreakpointsForDimension1=cumulative_dist_along_path  Table=path_y  ExtrapMethod=Clip  DiagnosticForOutOfRangeInput=Error  InternalRulePriority=Speed  RndMeth=Simplest  InputSameDT=on
  Atan2 : Trigonometry  Operator=atan2
  Derivative : Derivative
  Derivative1 : Derivative
  Scope : Scope
  Unwrap : dspsigops/Unwrap  tol=pi  InputProcessing=Columns as channels (frame based)  running=off
  Zero-Order Hold : ZeroOrderHold  SampleTime=-1
  X_sigma : Outport
  Y_sigma : Outport  Port=2
  psi_sigma : Outport  Port=3
  wires:
  total travelled distance/1 -> 1-D Lookup Table1/1, 1-D Lookup Table/1
  Unwrap/1 -> Scope/1, psi_sigma/1
  1-D Lookup Table/1 -> X_sigma/1, Derivative1/1  "interpolated path x value"
  Derivative1/1 -> Atan2/2  "dx"
  Derivative/1 -> Atan2/1  "dy"
  Atan2/1 -> Zero-Order Hold/1
  1-D Lookup Table1/1 -> Y_sigma/1, Derivative/1  "interpolated path y value"
  Zero-Order Hold/1 -> Unwrap/1

== system bike_model_v1_20190513_oldmodel/Path Tracking Controllers/Reference Position and Direction in Global CS with variable Look Ahead/Subsystem1 ==
  total travelled distance : Inport
  1-D Lookup Table : Lookup_n-D  NumberOfTableDimensions=1  BreakpointsForDimension1=cumulative_dist_along_path  Table=path_x  ExtrapMethod=Clip  DiagnosticForOutOfRangeInput=Error  InternalRulePriority=Speed  RndMeth=Simplest  InputSameDT=on
  1-D Lookup Table1 : Lookup_n-D  NumberOfTableDimensions=1  BreakpointsForDimension1=cumulative_dist_along_path  Table=path_y  ExtrapMethod=Clip  DiagnosticForOutOfRangeInput=Error  InternalRulePriority=Speed  RndMeth=Simplest  InputSameDT=on
  Atan2 : Trigonometry  Operator=atan2
  Derivative : Derivative
  Derivative1 : Derivative
  Scope : Scope
  Unwrap : dspsigops/Unwrap  tol=pi  InputProcessing=Columns as channels (frame based)  running=off
  Zero-Order Hold : ZeroOrderHold  SampleTime=-1
  X_sigma : Outport
  Y_sigma : Outport  Port=2
  psi_sigma : Outport  Port=3
  wires:
  total travelled distance/1 -> 1-D Lookup Table1/1, 1-D Lookup Table/1
  Unwrap/1 -> Scope/1, psi_sigma/1
  1-D Lookup Table/1 -> X_sigma/1, Derivative1/1  "interpolated path x value"
  Derivative1/1 -> Atan2/2  "dx"
  Derivative/1 -> Atan2/1  "dy"
  Atan2/1 -> Zero-Order Hold/1
  1-D Lookup Table1/1 -> Y_sigma/1, Derivative/1  "interpolated path y value"
  Zero-Order Hold/1 -> Unwrap/1
